simulink model "embeddedM_example"  (R2024b)
settings: Solver=FixedStepDiscrete  StartTime=0.0  StopTime=10.0  FixedStep=Ts  RelTol=1e-3
undefined symbols (not defined in the file): Ad, Bd, Cd, Dd
libraries: simulink x1
settings Model: Creator=wolfgang  LastModifiedBy=Amar
settings SolverCC: AlgebraicLoopSolver=TrustRegion
settings DataIOCC: ReturnWorkspaceOutputs=off
settings DebuggingCC: UnconnectedInputMsg=warning  UnconnectedOutputMsg=warning  UnconnectedLineMsg=warning  ArithmeticOperatorsInVariantConditions=warning
settings ModelReferenceCC: EnableRefExpFcnMdlSchedulingChecks=on
settings SFSimCC: SimUseLocalCustomCode=off  CustomCodeUndefinedFunction=UseInterfaceOnly
settings RTWCC: RTWUseLocalCustomCode=off  GPUComputeCapability=3.5

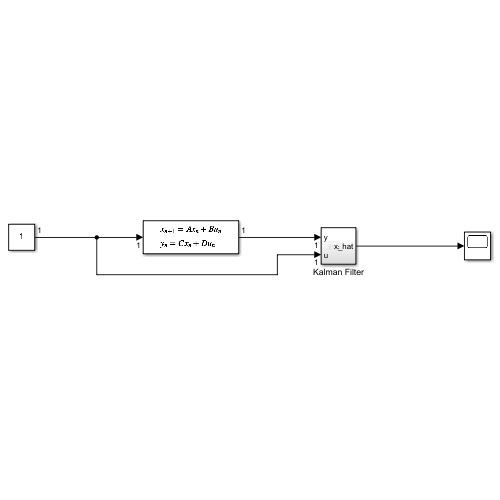
[thumbnail: Simulink's stored preview of the top-level diagram]
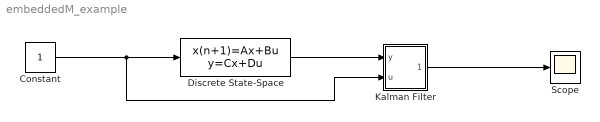
== system embeddedM_example ==
  Constant : Constant
  Discrete State-Space : DiscreteStateSpace  A=Ad  B=Bd  C=Cd  D=Dd  SampleTime=-1
  Kalman Filter : Subsystem
  Scope : Scope
  wires:
  Discrete State-Space/1 -> Kalman Filter/1(y)
  Constant/1 -> Kalman Filter/2(u), Discrete State-Space/1
  Kalman Filter/1(x_hat) -> Scope/1

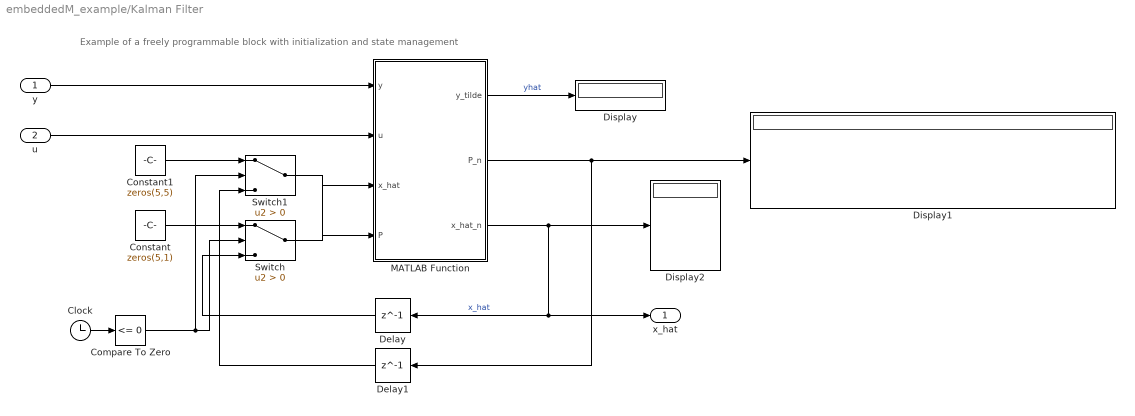
== system embeddedM_example/Kalman Filter ==
  note: Example of a freely programmable block with initialization and state management
  y : Inport
  u : Inport  Port=2
  Clock : Clock
  Compare To Zero : simulink/Logic and Bit Operations/Compare To Zero  relop=<=  OutDataTypeStr=boolean
  Constant : Constant  Value=zeros(5,1)
  Constant1 : Constant  Value=zeros(5,5)
  Delay : Delay  DelayLength=1  InitialCondition=0  SampleTime=1
  Delay1 : Delay  DelayLength=1  InitialCondition=0  SampleTime=1
  Display : Display
  Display1 : Display
  Display2 : Display
  MATLAB Function : MATLAB Function  TreatAsAtomicUnit=on
  Switch : Switch  Criteria=u2 > Threshold  SaturateOnIntegerOverflow=off  InputSameDT=off
  Switch1 : Switch  Criteria=u2 > Threshold  SaturateOnIntegerOverflow=off  InputSameDT=off
  x_hat : Outport
  wires:
  Delay/1 -> Switch/3
  Switch/1 -> MATLAB Function/3(x_hat)
  Constant1/1 -> Switch1/1
  Compare To Zero/1 -> Switch1/2, Switch/2
  MATLAB Function/3(x_hat_n) -> Display2/1, x_hat/1, Delay/1  "x_hat"
  Constant/1 -> Switch/1
  MATLAB Function/1(y_tilde) -> Display/1  "yhat"
  MATLAB Function/2(P_n) -> Display1/1, Delay1/1
  Clock/1 -> Compare To Zero/1
  Switch1/1 -> MATLAB Function/4(P)
  y/1 -> MATLAB Function/1(y)
  Delay1/1 -> Switch1/3
  u/1 -> MATLAB Function/2(u)

== matlab function embeddedM_example/Kalman Filter/MATLAB Function ==
  data: y input; u input; x_hat input; y_tilde output; P input; P_n output; x_hat_n output
function [y_tilde,P_n,x_hat_n] = fcn(y,u,x_hat,P)

% Predict
x_hat_n = Ad*x_hat + Bd*u
P_n = Ad*P*Ad' + Q

% Update
y_tilde = y - Cd*x_hat
x_hat_n = x_hat_n + K*y_tilde
P_n = (eye(2) - K*Cd)*P_n
y_tilde = y - Ad*x_hat_n
